simulink model "enable_disable"  (R2025b)
settings: Solver=FixedStepDiscrete  StartTime=0.0  StopTime=10  FixedStep=0.01  RelTol=1e-3
libraries: simulink x1
settings Model: Creator=Educação  LastModifiedBy=mateu

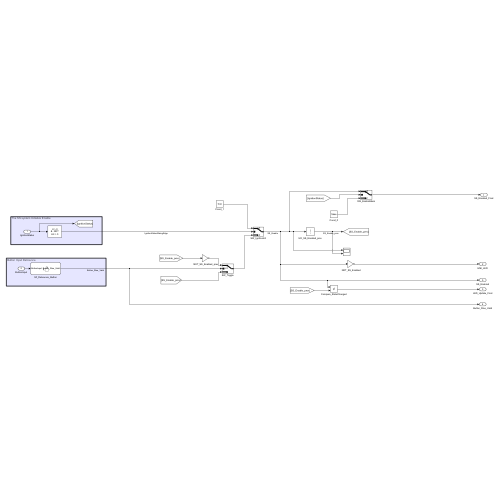
[thumbnail: Simulink's stored preview of the top-level diagram]
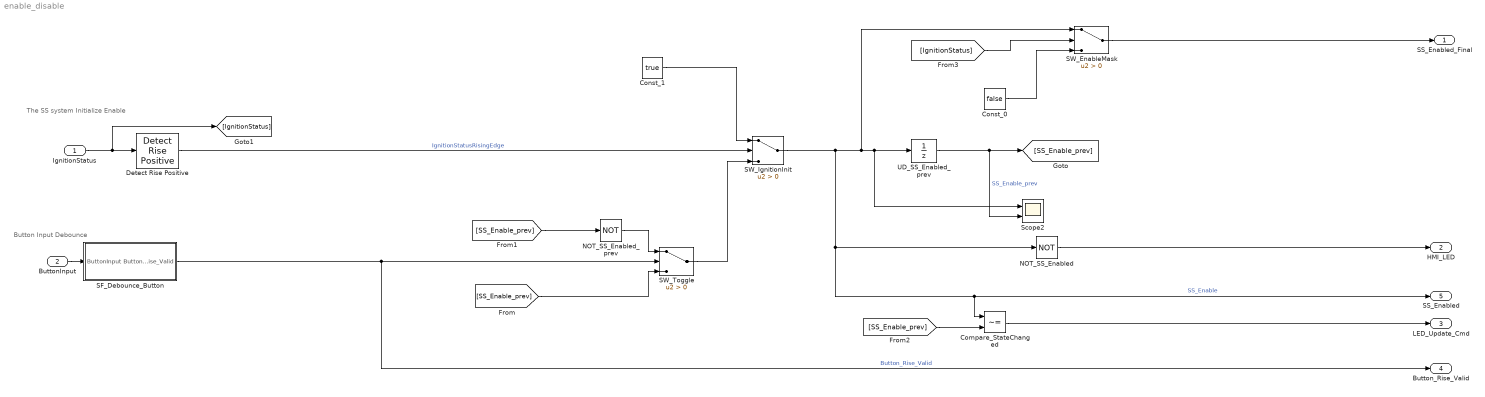
== system enable_disable ==
  note: Button Input Debounce
  note: The SS system Initialize Enable
  IgnitionStatus : Inport  OutDataTypeStr=boolean
  ButtonInput : Inport  Port=2  OutDataTypeStr=boolean
  Compare_StateChanged : RelationalOperator  Operator=~=  OutDataTypeStr=boolean  RndMeth=Simplest  InputSameDT=off
  Const_0 : Constant  Value=false
  Const_1 : Constant  Value=true
  Detect Rise Positive : simulink/Logic and Bit Operations/Detect Rise Positive  vinit=0  OutDataTypeStr=boolean
  NOT_SS_Enabled : Logic  Operator=NOT  IconShape=distinctive  AllPortsSameDT=off  OutDataTypeStr=boolean
  NOT_SS_Enabled_prev : Logic  Operator=NOT  IconShape=distinctive  AllPortsSameDT=off  OutDataTypeStr=boolean
  SF_Debounce_Button : Stateflow chart  TreatAsAtomicUnit=on
  SW_EnableMask : Switch  Criteria=u2 > Threshold  SaturateOnIntegerOverflow=off  InputSameDT=off
  SW_IgnitionInit : Switch  Criteria=u2 > Threshold  SaturateOnIntegerOverflow=off  InputSameDT=off
  SW_Toggle : Switch  Criteria=u2 > Threshold  SaturateOnIntegerOverflow=off  InputSameDT=off
  Scope2 : Scope  NumInputPorts=2
      settings: ActiveDisplayYMinimum=-0.125  ActiveDisplayYMaximum=1.125  DataLoggingVariableName=ScopeData3
  UD_SS_Enabled_prev : UnitDelay  InitialCondition=false  SampleTime=-1  HasFrameUpgradeWarning=on
  SS_Enabled_Final : Outport
  HMI_LED : Outport  Port=2
  LED_Update_Cmd : Outport  Port=3
  Button_Rise_Valid : Outport  Port=4
  SS_Enabled : Outport  Port=5
  wires:
  NOT_SS_Enabled_prev/1 -> SW_Toggle/1
  Detect Rise Positive/1 -> SW_IgnitionInit/2  "IgnitionStatusRisingEdge"
  [SS_Enable_prev] -> NOT_SS_Enabled_prev/1
  [SS_Enable_prev] -> Compare_StateChanged/2
  [SS_Enable_prev] -> SW_Toggle/3
  Const_1/1 -> SW_IgnitionInit/1
  Compare_StateChanged/1 -> LED_Update_Cmd/1
  SW_Toggle/1 -> SW_IgnitionInit/3
  NOT_SS_Enabled/1 -> HMI_LED/1
  IgnitionStatus/1 -> [IgnitionStatus], Detect Rise Positive/1
  Const_0/1 -> SW_EnableMask/3
  UD_SS_Enabled_prev/1 -> Scope2/2, [SS_Enable_prev]  "SS_Enable_prev"
  SW_IgnitionInit/1 -> NOT_SS_Enabled/1, Compare_StateChanged/1, SS_Enabled/1, SW_EnableMask/1, UD_SS_Enabled_prev/1, Scope2/1  "SS_Enable"
  ButtonInput/1 -> SF_Debounce_Button/1(ButtonInput)
  SW_EnableMask/1 -> SS_Enabled_Final/1
  SF_Debounce_Button/1(Button_Rise_Valid) -> Button_Rise_Valid/1, SW_Toggle/2  "Button_Rise_Valid"
  [IgnitionStatus] -> SW_EnableMask/2

== stateflow chart enable_disable/SF_Debounce_Button ==
  state Idle
    entry:
    Button_Rise_Valid = 0;
  state Debouncing
    entry:
    Button_Rise_Valid = 0;
  state Pressed
    entry:
    Button_Rise_Valid = 1;
  state WaitRelease
    entry:
    Button_Rise_Valid = 0;
  (default) -> Idle
  WaitRelease -> Idle : [ButtonInput == 0]
  Debouncing -> Idle [order 2] : [ButtonInput == 0]
  Idle -> Debouncing : [ButtonInput == 1]
  Debouncing -> Pressed [order 1] : [after(5, tick) && ButtonInput == 1]
  Pressed -> WaitRelease
  data: ButtonInput input; Button_Rise_Valid output
